simulink model "paper_model_20230707"  (R2022a)
settings: Solver=ode4  StartTime=0.0  StopTime=0.196  FixedStep=0.0001  RelTol=1e-3  AbsTol=1e-6
undefined symbols (not defined in the file or in its folder): contrapulset0, contrapulset1, contrastimrate, ipsipulset0, ipsipulset1, ipsistimrate, MaxEBNfr, opnThresholdBias, tauEBN, tauOPN, wEbnPlant, wErrorRate, wFbintLlbn, wIbnOpn, wIntPlant, wOpnEbn, wSlidePlant
settings Model: Creator=robi  LastModifiedBy=robi
settings DataIOCC: SaveFormat=Array  SignalLoggingSaveFormat=ModelDataLogs  ReturnWorkspaceOutputs=off
settings OptimizationCC: BlockReduction=off  BooleanDataType=off
settings DebuggingCC: SaveWithParameterizedLinksMsg=none  UnderspecifiedInitializationDetection=Classic  MergeDetectMultiDrivingBlocksExec=none  SignalResolutionControl=TryResolveAllWithWarning  InheritedTsInSrcMsg=none  MultiTaskDSMMsg=warning  MultiTaskCondExecSysMsg=none  UnconnectedInputMsg=warning  UnconnectedOutputMsg=warning  UnconnectedLineMsg=warning
settings HardwareCC: TargetUnknown=on
settings ModelReferenceCC: PropagateSignalLabelsOutOfModel=off
settings GRTTargetCC: TargetFcnLib=ansi_tfl_tmw.mat  TargetLangStandard=C89/C90 (ANSI)  CombineOutputUpdateFcns=off  GRTInterface=on
settings ConfigComp: CovMetricSettings=dw  CovSaveCumulativeToWorkspaceVar=on  CovSaveSingleToWorkspaceVar=on

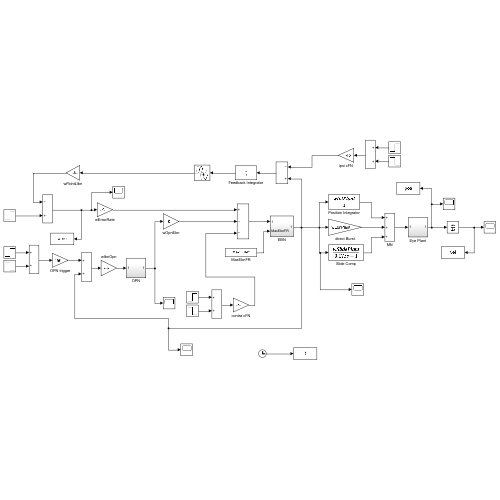
[thumbnail: Simulink's stored preview of the top-level diagram]
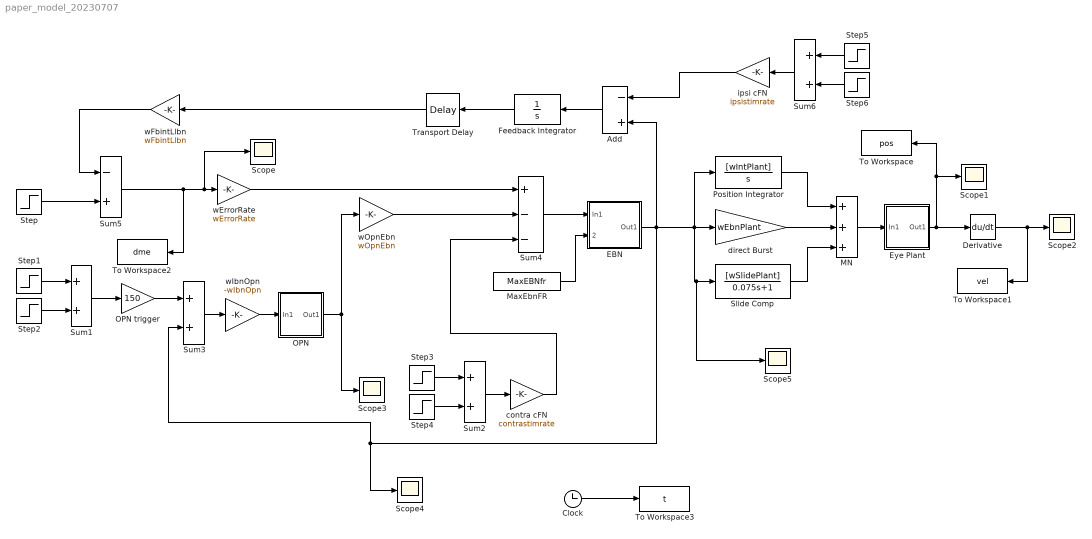
== system paper_model_20230707 ==
  Add : Sum  Inputs=-+
  Clock : Clock
  Derivative : Derivative
  EBN : Subsystem
  Eye Plant : Subsystem
  Feedback Integrator : TransferFcn  Denominator=[1 0]
  MN : Sum  Inputs=+++  InputSameDT=on  SaturateOnIntegerOverflow=on  OutDataTypeStr=Inherit: Same as first input
  MaxEbnFR : Constant  Value=MaxEBNfr
  OPN : Subsystem
  OPN trigger : Gain  Gain=150  SaturateOnIntegerOverflow=on  OutDataTypeStr=Inherit: Same as input  ParamDataTypeStr=Inherit: Same as input
  Position Integrator : TransferFcn  Numerator=[wIntPlant]  Denominator=[1 0]
  Scope{,1..5} (6 alike) : Scope
  Slide Comp : TransferFcn  Numerator=[wSlidePlant]  Denominator=[0.075 1]
  Step : Step  Time=0  After=24
  Step1 : Step  Time=0.04  SampleTime=0
  Step2 : Step  Time=0.05  After=-1  SampleTime=0
  Step3 : Step  Time=contrapulset0  SampleTime=0
  Step4 : Step  Time=contrapulset1  After=-1  SampleTime=0
  Step5 : Step  Time=ipsipulset0  SampleTime=0
  Step6 : Step  Time=ipsipulset1  After=-1  SampleTime=0
  Sum{1..3,6} (4 alike) : Sum  InputSameDT=on  SaturateOnIntegerOverflow=on  OutDataTypeStr=Inherit: Same as first input
  Sum4 : Sum  Inputs=+--  InputSameDT=on  SaturateOnIntegerOverflow=on  OutDataTypeStr=Inherit: Same as first input
  Sum5 : Sum  Inputs=-+  InputSameDT=on  SaturateOnIntegerOverflow=on  OutDataTypeStr=Inherit: Same as first input
  To Workspace : ToWorkspace  VariableName=pos  SampleTime=-1
  To Workspace1 : ToWorkspace  VariableName=vel  SampleTime=-1
  To Workspace2 : ToWorkspace  VariableName=dme  SampleTime=-1
  To Workspace3 : ToWorkspace  VariableName=t  SampleTime=-1
  Transport Delay : TransportDelay  DelayTime=0.005
  contra cFN : Gain  Gain=contrastimrate  SaturateOnIntegerOverflow=on  OutDataTypeStr=Inherit: Same as input  ParamDataTypeStr=Inherit: Same as input
  direct Burst : Gain  Gain=wEbnPlant  SaturateOnIntegerOverflow=on  OutDataTypeStr=Inherit: Same as input  ParamDataTypeStr=Inherit: Same as input
  ipsi cFN : Gain  Gain=ipsistimrate  SaturateOnIntegerOverflow=on  OutDataTypeStr=Inherit: Same as input  ParamDataTypeStr=Inherit: Same as input
  wErrorRate : Gain  Gain=wErrorRate  SaturateOnIntegerOverflow=on  OutDataTypeStr=Inherit: Same as input  ParamDataTypeStr=Inherit: Same as input
  wFbintLlbn : Gain  Gain=wFbintLlbn  SaturateOnIntegerOverflow=on  OutDataTypeStr=Inherit: Same as input  ParamDataTypeStr=Inherit: Same as input
  wIbnOpn : Gain  Gain=-wIbnOpn  SaturateOnIntegerOverflow=on  OutDataTypeStr=Inherit: Same as input  ParamDataTypeStr=Inherit: Same as input
  wOpnEbn : Gain  Gain=wOpnEbn  SaturateOnIntegerOverflow=on  OutDataTypeStr=Inherit: Same as input  ParamDataTypeStr=Inherit: Same as input
  wires:
  MN/1 -> Eye Plant/1(In1)
  Position Integrator/1 -> MN/1
  direct Burst/1 -> MN/2
  Slide Comp/1 -> MN/3
  Sum4/1 -> EBN/1(In1)
  Sum5/1 -> To Workspace2/1, wErrorRate/1, Scope/1
  wFbintLlbn/1 -> Sum5/1
  MaxEbnFR/1 -> EBN/2(MaxEbnFR)
  Step/1 -> Sum5/2
  wOpnEbn/1 -> Sum4/2
  Eye Plant/1(Out1) -> Derivative/1, To Workspace/1, Scope1/1
  OPN/1(Out1) -> Scope3/1, wOpnEbn/1
  Feedback Integrator/1 -> Transport Delay/1
  Transport Delay/1 -> wFbintLlbn/1
  wErrorRate/1 -> Sum4/1
  Step1/1 -> Sum1/1
  Step2/1 -> Sum1/2
  Sum1/1 -> OPN trigger/1
  OPN trigger/1 -> Sum3/1
  EBN/1(Out1) -> Sum3/2, Scope4/1, Add/2, Scope5/1, Slide Comp/1, Position Integrator/1, direct Burst/1
  Step3/1 -> Sum2/1
  Step4/1 -> Sum2/2
  Sum2/1 -> contra cFN/1
  contra cFN/1 -> Sum4/3
  Add/1 -> Feedback Integrator/1
  Step5/1 -> Sum6/1
  Sum6/1 -> ipsi cFN/1
  Step6/1 -> Sum6/2
  ipsi cFN/1 -> Add/1
  Derivative/1 -> To Workspace1/1, Scope2/1
  Sum3/1 -> wIbnOpn/1
  wIbnOpn/1 -> OPN/1(In1)
  Clock/1 -> To Workspace3/1

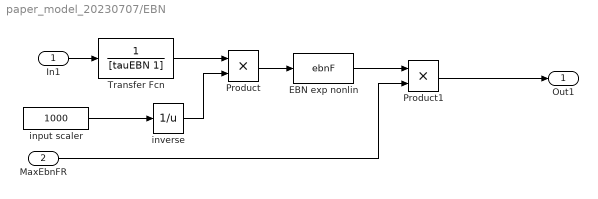
== system paper_model_20230707/EBN ==
  In1 : Inport
  MaxEbnFR : Inport  Port=2
  EBN exp nonlin : MATLABFcn  MATLABFcn=ebnF
  Product : Product  InputSameDT=on  RndMeth=Zero  SaturateOnIntegerOverflow=on  OutDataTypeStr=Inherit: Same as first input
  Product1 : Product  Inputs=**  InputSameDT=on  RndMeth=Zero  SaturateOnIntegerOverflow=on  OutDataTypeStr=Inherit: Same as first input
  Transfer Fcn : TransferFcn  Denominator=[tauEBN 1]
  input scaler : Constant  Value=1000
  inverse : Math  Operator=reciprocal  SignedPower=on
  Out1 : Outport
  wires:
  In1/1 -> Transfer Fcn/1
  Product/1 -> EBN exp nonlin/1
  Transfer Fcn/1 -> Product/1
  EBN exp nonlin/1 -> Product1/1
  Product1/1 -> Out1/1
  inverse/1 -> Product/2
  MaxEbnFR/1 -> Product1/2
  input scaler/1 -> inverse/1

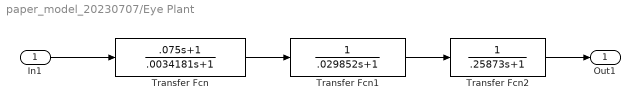
== system paper_model_20230707/Eye Plant ==
  In1 : Inport
  Transfer Fcn : TransferFcn  Numerator=[.075 1]  Denominator=[.0034181 1]
  Transfer Fcn1 : TransferFcn  Denominator=[.029852 1]
  Transfer Fcn2 : TransferFcn  Denominator=[.25873 1]
  Out1 : Outport
  wires:
  Transfer Fcn/1 -> Transfer Fcn1/1
  Transfer Fcn1/1 -> Transfer Fcn2/1
  Transfer Fcn2/1 -> Out1/1
  In1/1 -> Transfer Fcn/1

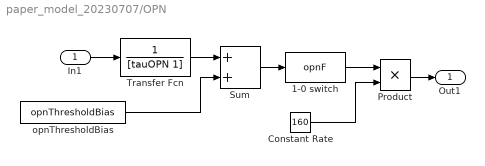
== system paper_model_20230707/OPN ==
  In1 : Inport
  1-0 switch : MATLABFcn  MATLABFcn=opnF
  Constant Rate : Constant  Value=160
  Product : Product  Inputs=**  InputSameDT=on  RndMeth=Zero  SaturateOnIntegerOverflow=on  OutDataTypeStr=Inherit: Same as first input
  Sum : Sum  InputSameDT=on  SaturateOnIntegerOverflow=on  OutDataTypeStr=Inherit: Same as first input
  Transfer Fcn : TransferFcn  Denominator=[tauOPN 1]
  opnThresholdBias : Constant  Value=opnThresholdBias
  Out1 : Outport
  wires:
  In1/1 -> Transfer Fcn/1
  Transfer Fcn/1 -> Sum/1
  opnThresholdBias/1 -> Sum/2
  Sum/1 -> 1-0 switch/1
  1-0 switch/1 -> Product/1
  Constant Rate/1 -> Product/2
  Product/1 -> Out1/1
